simulink model "3_3PVstring"  (R2023b)
settings: Solver=ode3  StartTime=0.0  StopTime=1  FixedStep=1e-5  RelTol=1e-3
libraries: spsDiodeLib x18, spsPVArrayLib x9, spsIGBTDiodeLib x6, spsSeriesRLCBranchLib x3, spsSawtoothGeneratorLib x3, spsVoltageMeasurementLib x2, spsGroundLib x1, spsThreePhaseVIMeasurementLib x1, spsControlledVoltageSourceLib x1, spsCurrentMeasurementLib x1, simulink x1, sps_lib x1
settings Model: Creator=ameen  LastModifiedBy=safad

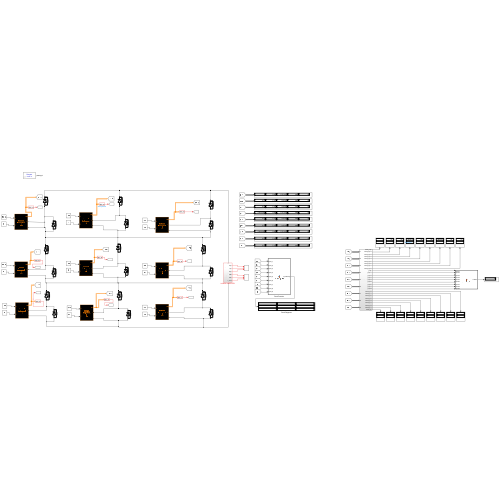
[thumbnail: Simulink's stored preview of the top-level diagram]
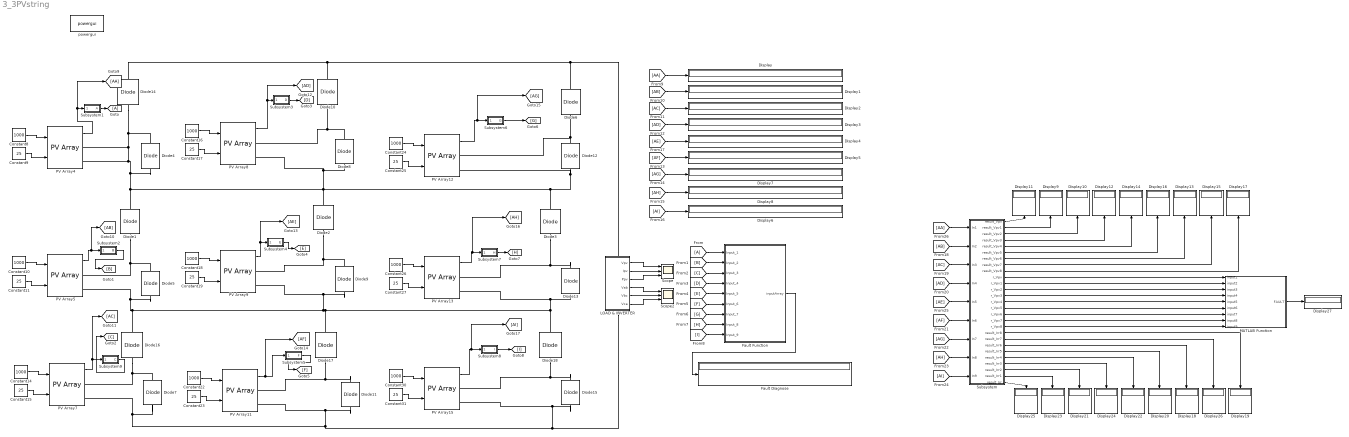
== system 3_3PVstring ==
  Constant{8,10,14,16,18,22,24,26,30} (9 alike) : Constant  Value=1000
  Constant{9,11,15,17,19,23,25,27,31} (9 alike) : Constant  Value=25
  Diode{1..18} (18 alike) : spsDiodeLib/Diode  Ron=0.001  Lon=0  Vf=0.8  IC=0  UseSnubber=0  Rs=500  Cs=250e-9  Measurements=off
  Display{,1..27} (28 alike) : Display
  Fault Diagnose : Display
  Fault Function : MATLAB Function  TreatAsAtomicUnit=on
  From : From
  Goto : Goto
  LOAD & INVERTER : Subsystem
      settings: PortSchema="{\"entries\":[{\"content\":{\"sides\":[{\"content\":{},\"type\":\"ConnectorPlacement.EquallySpacedRectSide\",\"uuid\":\"9d5a924a-1d3a-4741-a2b7-92be7c614fd7\"},{\"content\":{\"connectorIds\":[\"Out1\",\"Out2\",\"Out3\",\"Out4\",\"Out5\",\"Out6\"],\"side\":\"RIGHT\"},\"type\":\"ConnectorPlacement.EquallySpacedRectSide\",\"uuid\":\"42e89420-eace-4661-8437-77e02d17d38a\"},{\"content\":{\"connectorIds\":[\"LConn1\"],\"side\":\"TOP\"},\"type\":\"ConnectorPlacement.EquallySpacedRectSide\",\"uuid\":\"88a88f09-a234-44ff-a45c-243ed75cbb49\"},{\"content\":{\"connectorIds\":[\"RConn1\"],\"side\":\"BOTTOM\"},\"type\":\"ConnectorPlacement.EquallySpacedRectSide\",\"uuid\":\"b84592b4-f439-4f10-a620-72ac78255a9b\"}]},\"type\":\"ConnectorPlacement.EquallySpacedConnector\",\"uuid\":\"5a103a7e-397f-4ab8-8786-2dccd824124f\"}],\"packageUris\":[\"http://schema.mathworks.com/mf0/Connector/R2020b\"],\"version\":\"1.0\"}"
  MATLAB Function : MATLAB Function  TreatAsAtomicUnit=on
  PV Array{4..5,7..9,11..13,15} (9 alike) : spsPVArrayLib/PV Array  Npar=1  Nser=1  PlotType=array @ 25 deg.C & specified irradiances  S_vec="[ 1000  500  100 ]"  Temp_C_vec="[ 45 25  ]"  ModuleName=User-defined  PlotWhenSelected=off  Pm=213.15  Ncell=60  Voc=36.3  Isc=7.84  Vm=29  Im=7.35  beta_Voc_pc=-0.36099  alpha_Isc_pc=0.102  beta_Voc=-0.13104  alpha_Isc=0.0079968  IL=7.8654  I0=2.9273e-10  nI=0.98119  Rsh=313.0553  Rs=0.39381  RobustModel=off  RobustCellTemperature=313.3991  BAL=off  Tc=1e-6  Tfilter=1e-5
  Scope : Scope  NumInputPorts=3
  Scope2 : Scope  NumInputPorts=3
  Subsystem : Subsystem
  Subsystem1 : Subsystem
  Subsystem2 : Subsystem
  Subsystem3 : Subsystem
  Subsystem4 : Subsystem
  Subsystem5 : Subsystem
  Subsystem6 : Subsystem
  Subsystem7 : Subsystem
  Subsystem8 : Subsystem
  Subsystem9 : Subsystem
  powergui : sps_lib/powergui  Priority=1  SimulationMode=Discrete  SampleTime=1e-5  frequency=60  Iterations=50  frequencyindice=0  Pbase=100e6  ErrMax=1e-4  UnitsV=kV  UnitsW=MW  buscounter=0  FunctionMessages=off  echomessages=off  EnableUseOfTLC=off  CurrentSourceSwitches=off  DisableSnubberDevices=off  DisableRonSwitches=off  DisableVfSwitches=off  DisplayEquations=off  AutomaticDiscreteSolvers=off  SolverType=Tustin  Interpol=off  ExternalGateDelay=off  methode=off  Ts=100  x0status=blocks  SPID=on  SwTol=0  HookPort=off  NonlinearTolerance=1e-4  nMaxIteration=100  ContinueOnMaxIteration=off  RestoreLinks=warning  ResistiveCurrentMeasurement=off  Frange=[0:2:500]  Ylog=off  Xlog=on  ShowGrid=off  save=off  variable=ZData  structure=0  ZoomFFT=off  StartTime=0.0  cycles=1  DisplayStyle=1  fundamental=60  FreqAxis=off  MaxFrequency=1000  frequencyindicesteady=1  RmsSteady=1  display=off
  wires:
  Constant15/1 -> PV Array7/2
  Constant14/1 -> PV Array7/1
  Constant11/1 -> PV Array5/2
  Constant9/1 -> PV Array4/2
  Constant8/1 -> PV Array4/1
  Constant10/1 -> PV Array5/1
  Constant23/1 -> PV Array11/2
  Constant22/1 -> PV Array11/1
  Constant19/1 -> PV Array9/2
  Constant17/1 -> PV Array8/2
  Constant16/1 -> PV Array8/1
  Constant18/1 -> PV Array9/1
  Constant31/1 -> PV Array15/2
  Constant30/1 -> PV Array15/1
  Constant27/1 -> PV Array13/2
  Constant25/1 -> PV Array12/2
  Constant24/1 -> PV Array12/1
  Constant26/1 -> PV Array13/1
  PV Array4/1 -> [AA], Subsystem1/1(Vpv)
  Subsystem1/1(A) -> Goto/1
  Subsystem3/1(D) -> [D]
  PV Array8/1 -> [AD], Subsystem3/1(Vpv)
  PV Array12/1 -> [AG], Subsystem6/1(Vpv)
  Subsystem6/1(G) -> [G]
  Subsystem2/1(B) -> [B]
  PV Array5/1 -> [AB], Subsystem2/1(Vpv)
  PV Array9/1 -> [AE], Subsystem4/1(Vpv)
  Subsystem4/1(E) -> [E]
  Subsystem5/1(F) -> [F]
  PV Array11/1 -> [AF], Subsystem5/1(Vpv)
  Subsystem7/1(H) -> [H]
  PV Array13/1 -> [AH], Subsystem7/1(Vpv)
  Subsystem8/1(I) -> [I]
  PV Array15/1 -> [AI], Subsystem8/1(Vpv)
  [D] -> Fault Function/4(Input_4)
  [B] -> Fault Function/2(Input_2)
  [F] -> Fault Function/6(Input_6)
  [E] -> Fault Function/5(Input_5)
  [G] -> Fault Function/7(Input_7)
  Fault Function/1(inputArray) -> Fault Diagnose/1
  [C] -> Fault Function/3(Input_3)
  [I] -> Fault Function/9(Input_9)
  [H] -> Fault Function/8(Input_8)
  From/1 -> Fault Function/1(Input_1)
  PV Array7/1 -> [AC], Subsystem9/1(Vpv)
  Subsystem9/1(C) -> [C]
  LOAD & INVERTER/1(Vpv) -> Scope/1
  LOAD & INVERTER/2(Ipv) -> Scope/2
  LOAD & INVERTER/3(Ppv) -> Scope/3
  LOAD & INVERTER/4(Vab) -> Scope2/1
  LOAD & INVERTER/5(Vbc) -> Scope2/2
  LOAD & INVERTER/6(Vca) -> Scope2/3
  [AA] -> Display/1
  [AB] -> Display1/1
  [AC] -> Display2/1
  [AD] -> Display3/1
  [AE] -> Display4/1
  [AF] -> Display5/1
  [AG] -> Display7/1
  [AH] -> Display8/1
  [AI] -> Display6/1
  [AA] -> Subsystem/1(In1)
  [AB] -> Subsystem/2(In2)
  [AC] -> Subsystem/3(In3)
  [AD] -> Subsystem/4(In4)
  [AE] -> Subsystem/5(In5)
  [AF] -> Subsystem/6(In6)
  [AG] -> Subsystem/7(In7)
  [AH] -> Subsystem/8(In8)
  [AI] -> Subsystem/9(In9)
  Subsystem/1(result_Vpv) -> Display11/1
  Subsystem/2(result_Vpv1) -> Display9/1
  Subsystem/3(result_Vpv2) -> Display10/1
  Subsystem/4(result_Vpv3) -> Display12/1
  Subsystem/5(result_Vpv4) -> Display14/1
  Subsystem/6(result_Vpv5) -> Display16/1
  Subsystem/7(result_Vpv6) -> Display13/1
  Subsystem/8(result_Vpv7) -> Display15/1
  Subsystem/9(result_Vpv8) -> Display17/1
  Subsystem/27(result_Irr) -> Display25/1
  Subsystem/26(result_Irr1) -> Display23/1
  Subsystem/25(result_Irr2) -> Display21/1
  Subsystem/24(result_Irr3) -> Display24/1
  Subsystem/23(result_Irr4) -> Display22/1
  Subsystem/22(result_Irr5) -> Display20/1
  Subsystem/21(result_Irr6) -> Display18/1
  Subsystem/20(result_Irr7) -> Display26/1
  Subsystem/19(result_Irr8) -> Display19/1
  Subsystem/10(r_Vpv) -> MATLAB Function/1(input1)
  Subsystem/11(r_Vpv1) -> MATLAB Function/2(input2)
  Subsystem/12(r_Vpv2) -> MATLAB Function/3(input3)
  Subsystem/13(r_Vpv3) -> MATLAB Function/4(input4)
  Subsystem/14(r_Vpv4) -> MATLAB Function/5(input5)
  Subsystem/15(r_Vpv5) -> MATLAB Function/6(input6)
  Subsystem/16(r_Vpv6) -> MATLAB Function/7(input7)
  Subsystem/17(r_Vpv7) -> MATLAB Function/8(input8)
  Subsystem/18(r_Vpv8) -> MATLAB Function/9(input9)
  MATLAB Function/1(FAULT) -> Display27/1
  connections:
  Diode13/RConn1 -- Diode3/LConn1 -- PV Array13/RConn1
  Diode8/RConn1 -- Diode10/LConn1 -- PV Array8/RConn1
  Diode9/LConn1 -- Diode5/LConn1 -- PV Array5/RConn2 -- Diode16/RConn1 -- Diode17/RConn1 -- Diode13/LConn1 -- PV Array13/RConn2 -- Diode18/RConn1 -- PV Array9/RConn2
  Diode15/RConn1 -- Diode18/LConn1 -- PV Array15/RConn1
  Diode11/RConn1 -- Diode17/LConn1 -- PV Array11/RConn1
  Diode10/RConn1 -- Diode14/RConn1 -- Diode6/RConn1 -- LOAD & INVERTER/LConn1
  Diode1/LConn1 -- Diode5/RConn1 -- PV Array5/RConn1
  Diode16/LConn1 -- Diode7/RConn1 -- PV Array7/RConn1
  Diode12/RConn1 -- Diode6/LConn1 -- PV Array12/RConn1
  Diode11/LConn1 -- Diode7/LConn1 -- PV Array7/RConn2 -- LOAD & INVERTER/RConn1 -- Diode15/LConn1 -- PV Array15/RConn2 -- PV Array11/RConn2
  Diode9/RConn1 -- Diode2/LConn1 -- PV Array9/RConn1
  Diode14/LConn1 -- Diode4/RConn1 -- PV Array4/RConn2 -- Diode4/LConn1 -- Diode8/LConn1 -- PV Array8/RConn2 -- Diode2/RConn1 -- Diode12/LConn1 -- PV Array12/RConn2 -- Diode3/RConn1 -- Diode1/RConn1 -- PV Array4/RConn1

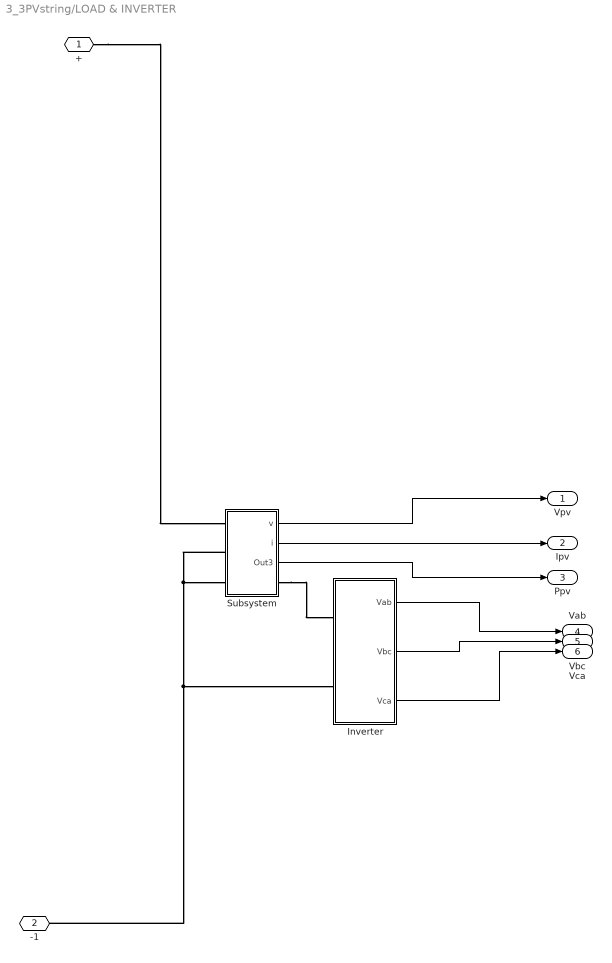
== system 3_3PVstring/LOAD & INVERTER ==
  Inverter : Subsystem
  Subsystem : Subsystem
  + : PMIOPort  Side=Left
  -1 : PMIOPort  Port=2  Side=Right
  Vpv : Outport
  Ipv : Outport  Port=2
  Ppv : Outport  Port=3
  Vab : Outport  Port=4
  Vbc : Outport  Port=5
  Vca : Outport  Port=6
  wires:
  Subsystem/1(v) -> Vpv/1
  Subsystem/2(i) -> Ipv/1
  Subsystem/3(Out3) -> Ppv/1
  Inverter/1(Vab) -> Vab/1
  Inverter/2(Vbc) -> Vbc/1
  Inverter/3(Vca) -> Vca/1
  connections:
  Subsystem/RConn1 -- Inverter/LConn1
  Subsystem/LConn2 -- -1/RConn1 -- Inverter/LConn2 -- Subsystem/LConn3
  +/RConn1 -- Subsystem/LConn1

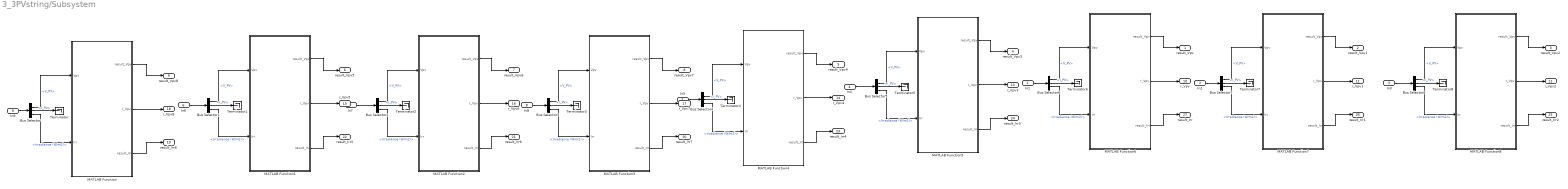
== system 3_3PVstring/Subsystem ==
  In1 : Inport
  In2 : Inport  Port=2
  In3 : Inport  Port=3
  In4 : Inport  Port=4
  In5 : Inport  Port=5
  In6 : Inport  Port=6
  In7 : Inport  Port=7
  In8 : Inport  Port=8
  In9 : Inport  Port=9
  Bus Selector{,1..8} (9 alike) : BusSelector  OutputSignals=V_PV,I_PV,Irradiance (W/m2)
  MATLAB Function : MATLAB Function  TreatAsAtomicUnit=on
  MATLAB Function1 : MATLAB Function  TreatAsAtomicUnit=on
  MATLAB Function2 : MATLAB Function  TreatAsAtomicUnit=on
  MATLAB Function3 : MATLAB Function  TreatAsAtomicUnit=on
  MATLAB Function4 : MATLAB Function  TreatAsAtomicUnit=on
  MATLAB Function5 : MATLAB Function  TreatAsAtomicUnit=on
  MATLAB Function6 : MATLAB Function  TreatAsAtomicUnit=on
  MATLAB Function7 : MATLAB Function  TreatAsAtomicUnit=on
  MATLAB Function8 : MATLAB Function  TreatAsAtomicUnit=on
  Terminator{,1..8} (9 alike) : Terminator
  result_Vpv : Outport
  result_Vpv1 : Outport  Port=2
  result_Vpv2 : Outport  Port=3
  result_Vpv3 : Outport  Port=4
  result_Vpv4 : Outport  Port=5
  result_Vpv5 : Outport  Port=6
  result_Vpv6 : Outport  Port=7
  result_Vpv7 : Outport  Port=8
  result_Vpv8 : Outport  Port=9
  r_Vpv : Outport  Port=10
  r_Vpv1 : Outport  Port=11
  r_Vpv2 : Outport  Port=12
  r_Vpv3 : Outport  Port=13
  r_Vpv4 : Outport  Port=14
  r_Vpv5 : Outport  Port=15
  r_Vpv6 : Outport  Port=16
  r_Vpv7 : Outport  Port=17
  r_Vpv8 : Outport  Port=18
  result_Irr8 : Outport  Port=19
  result_Irr7 : Outport  Port=20
  result_Irr6 : Outport  Port=21
  result_Irr5 : Outport  Port=22
  result_Irr4 : Outport  Port=23
  result_Irr3 : Outport  Port=24
  result_Irr2 : Outport  Port=25
  result_Irr1 : Outport  Port=26
  result_Irr : Outport  Port=27
  wires:
  MATLAB Function7/1(result_Vpv) -> result_Vpv1/1
  Bus Selector6/2 -> Terminator6/1  "<I_PV>"
  In3/1 -> Bus Selector8/1
  Bus Selector6/1 -> MATLAB Function6/1(Vpv)  "<V_PV>"
  Bus Selector/3 -> MATLAB Function/2(Irr)  "<Irradiance (W/m2)>"
  MATLAB Function8/1(result_Vpv) -> result_Vpv2/1
  Bus Selector1/3 -> MATLAB Function1/2(Irr)  "<Irradiance (W/m2)>"
  Bus Selector/1 -> MATLAB Function/1(Vpv)  "<V_PV>"
  MATLAB Function3/1(result_Vpv) -> result_Vpv7/1
  MATLAB Function8/2(r_Vpv) -> r_Vpv2/1
  In7/1 -> Bus Selector2/1
  MATLAB Function2/1(result_Vpv) -> result_Vpv6/1
  MATLAB Function6/1(result_Vpv) -> result_Vpv/1
  Bus Selector/2 -> Terminator/1  "<I_PV>"
  Bus Selector7/1 -> MATLAB Function7/1(Vpv)  "<V_PV>"
  MATLAB Function3/3(result_Irr) -> result_Irr7/1
  Bus Selector2/2 -> Terminator2/1  "<I_PV>"
  Bus Selector6/3 -> MATLAB Function6/2(Irr)  "<Irradiance (W/m2)>"
  In4/1 -> Bus Selector5/1
  MATLAB Function6/3(result_Irr) -> result_Irr/1
  MATLAB Function7/3(result_Irr) -> result_Irr1/1
  MATLAB Function/2(r_Vpv) -> r_Vpv8/1
  Bus Selector1/1 -> MATLAB Function1/1(Vpv)  "<V_PV>"
  Bus Selector7/3 -> MATLAB Function7/2(Irr)  "<Irradiance (W/m2)>"
  MATLAB Function5/3(result_Irr) -> result_Irr3/1
  Bus Selector4/3 -> MATLAB Function4/2(Irr)  "<Irradiance (W/m2)>"
  MATLAB Function1/2(r_Vpv) -> r_Vpv5/1
  MATLAB Function2/2(r_Vpv) -> r_Vpv6/1
  Bus Selector1/2 -> Terminator1/1  "<I_PV>"
  MATLAB Function3/2(r_Vpv) -> r_Vpv7/1
  Bus Selector3/2 -> Terminator3/1  "<I_PV>"
  In8/1 -> Bus Selector3/1
  Bus Selector3/1 -> MATLAB Function3/1(Vpv)  "<V_PV>"
  MATLAB Function8/3(result_Irr) -> result_Irr2/1
  Bus Selector3/3 -> MATLAB Function3/2(Irr)  "<Irradiance (W/m2)>"
  Bus Selector7/2 -> Terminator7/1  "<I_PV>"
  Bus Selector4/2 -> Terminator4/1  "<I_PV>"
  MATLAB Function2/3(result_Irr) -> result_Irr6/1
  MATLAB Function5/1(result_Vpv) -> result_Vpv3/1
  Bus Selector4/1 -> MATLAB Function4/1(Vpv)  "<V_PV>"
  Bus Selector2/3 -> MATLAB Function2/2(Irr)  "<Irradiance (W/m2)>"
  In1/1 -> Bus Selector6/1
  Bus Selector5/2 -> Terminator5/1  "<I_PV>"
  Bus Selector8/2 -> Terminator8/1  "<I_PV>"
  Bus Selector2/1 -> MATLAB Function2/1(Vpv)  "<V_PV>"
  In5/1 -> Bus Selector4/1
  Bus Selector8/1 -> MATLAB Function8/1(Vpv)  "<V_PV>"
  Bus Selector8/3 -> MATLAB Function8/2(Irr)  "<Irradiance (W/m2)>"
  In6/1 -> Bus Selector1/1
  MATLAB Function6/2(r_Vpv) -> r_Vpv/1
  MATLAB Function4/1(result_Vpv) -> result_Vpv4/1
  Bus Selector5/3 -> MATLAB Function5/2(Irr)  "<Irradiance (W/m2)>"
  MATLAB Function5/2(r_Vpv) -> r_Vpv3/1
  Bus Selector5/1 -> MATLAB Function5/1(Vpv)  "<V_PV>"
  MATLAB Function/3(result_Irr) -> result_Irr8/1
  MATLAB Function1/3(result_Irr) -> result_Irr5/1
  In9/1 -> Bus Selector/1
  MATLAB Function/1(result_Vpv) -> result_Vpv8/1
  MATLAB Function1/1(result_Vpv) -> result_Vpv5/1
  In2/1 -> Bus Selector7/1
  MATLAB Function7/2(r_Vpv) -> r_Vpv1/1
  MATLAB Function4/2(r_Vpv) -> r_Vpv4/1
  MATLAB Function4/3(result_Irr) -> result_Irr4/1

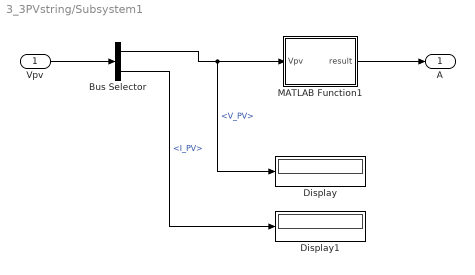
== system 3_3PVstring/Subsystem1 ==
  Vpv : Inport
  Bus Selector : BusSelector  OutputSignals=V_PV,I_PV
  Display : Display
  Display1 : Display
  MATLAB Function1 : MATLAB Function  TreatAsAtomicUnit=on
  A : Outport
  wires:
  Vpv/1 -> Bus Selector/1
  MATLAB Function1/1(result) -> A/1
  Bus Selector/1 -> Display/1, MATLAB Function1/1(Vpv)  "<V_PV>"
  Bus Selector/2 -> Display1/1  "<I_PV>"

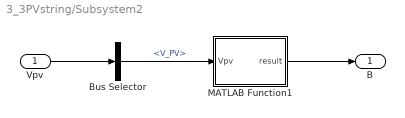
== system 3_3PVstring/Subsystem2 ==
  Vpv : Inport
  Bus Selector : BusSelector  OutputSignals=V_PV
  MATLAB Function1 : MATLAB Function  TreatAsAtomicUnit=on
  B : Outport
  wires:
  MATLAB Function1/1(result) -> B/1
  Vpv/1 -> Bus Selector/1
  Bus Selector/1 -> MATLAB Function1/1(Vpv)  "<V_PV>"

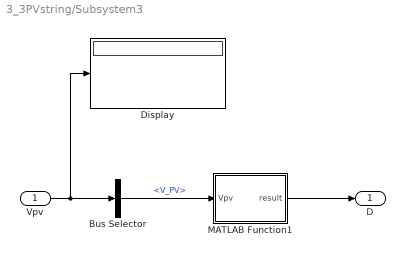
== system 3_3PVstring/Subsystem3 ==
  Vpv : Inport
  Bus Selector : BusSelector  OutputSignals=V_PV
  Display : Display
  MATLAB Function1 : MATLAB Function  TreatAsAtomicUnit=on
  D : Outport
  wires:
  MATLAB Function1/1(result) -> D/1
  Vpv/1 -> Bus Selector/1, Display/1
  Bus Selector/1 -> MATLAB Function1/1(Vpv)  "<V_PV>"

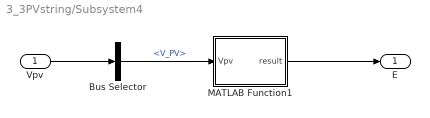
== system 3_3PVstring/Subsystem4 ==
  Vpv : Inport
  Bus Selector : BusSelector  OutputSignals=V_PV
  MATLAB Function1 : MATLAB Function  TreatAsAtomicUnit=on
  E : Outport
  wires:
  Bus Selector/1 -> MATLAB Function1/1(Vpv)  "<V_PV>"
  Vpv/1 -> Bus Selector/1
  MATLAB Function1/1(result) -> E/1

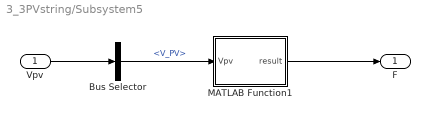
== system 3_3PVstring/Subsystem5 ==
  Vpv : Inport
  Bus Selector : BusSelector  OutputSignals=V_PV
  MATLAB Function1 : MATLAB Function  TreatAsAtomicUnit=on
  F : Outport
  wires:
  MATLAB Function1/1(result) -> F/1
  Vpv/1 -> Bus Selector/1
  Bus Selector/1 -> MATLAB Function1/1(Vpv)  "<V_PV>"

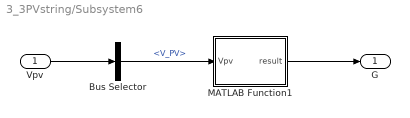
== system 3_3PVstring/Subsystem6 ==
  Vpv : Inport
  Bus Selector : BusSelector  OutputSignals=V_PV
  MATLAB Function1 : MATLAB Function  TreatAsAtomicUnit=on
  G : Outport
  wires:
  Bus Selector/1 -> MATLAB Function1/1(Vpv)  "<V_PV>"
  Vpv/1 -> Bus Selector/1
  MATLAB Function1/1(result) -> G/1

== system 3_3PVstring/Subsystem7 ==
  Vpv : Inport
  Bus Selector : BusSelector  OutputSignals=V_PV
  MATLAB Function1 : MATLAB Function  TreatAsAtomicUnit=on
  H : Outport
  wires:
  MATLAB Function1/1(result) -> H/1
  Vpv/1 -> Bus Selector/1
  Bus Selector/1 -> MATLAB Function1/1(Vpv)  "<V_PV>"

== system 3_3PVstring/Subsystem8 ==
  Vpv : Inport
  Bus Selector : BusSelector  OutputSignals=V_PV
  MATLAB Function1 : MATLAB Function  TreatAsAtomicUnit=on
  I : Outport
  wires:
  Bus Selector/1 -> MATLAB Function1/1(Vpv)  "<V_PV>"
  Vpv/1 -> Bus Selector/1
  MATLAB Function1/1(result) -> I/1

== system 3_3PVstring/Subsystem9 ==
  Vpv : Inport
  Bus Selector : BusSelector  OutputSignals=V_PV
  MATLAB Function1 : MATLAB Function  TreatAsAtomicUnit=on
  C : Outport
  wires:
  Bus Selector/1 -> MATLAB Function1/1(Vpv)  "<V_PV>"
  Vpv/1 -> Bus Selector/1
  MATLAB Function1/1(result) -> C/1

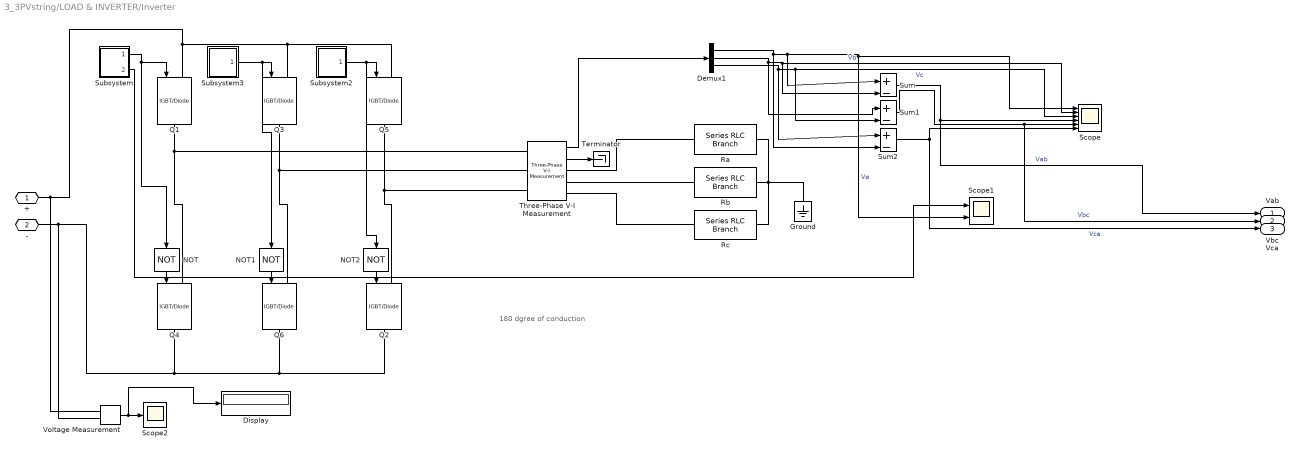
== system 3_3PVstring/LOAD & INVERTER/Inverter ==
  note: 180 dgree of conduction
  Demux1 : Demux  Outputs=3
  Display : Display
  Ground : spsGroundLib/Ground  LConnTagsString=a
  NOT : Logic  Operator=NOT  AllPortsSameDT=off  OutDataTypeStr=boolean
  NOT1 : Logic  Operator=NOT  AllPortsSameDT=off  OutDataTypeStr=boolean
  NOT2 : Logic  Operator=NOT  AllPortsSameDT=off  OutDataTypeStr=boolean
  Q{1..6} (6 alike) : spsIGBTDiodeLib/IGBT//Diode  Ron=1e-3  Rs=1e5  Cs=inf  Measurements=off
  Ra : spsSeriesRLCBranchLib/Series RLC Branch  LConnTagsString=__new0  RConnTagsString=__new0  BranchType=R  Resistance=-0.5820  Inductance=1e-3  SetiL0=off  InitialCurrent=0  Capacitance=1e-6  Setx0=off  InitialVoltage=0  Measurements=None
  Rb : spsSeriesRLCBranchLib/Series RLC Branch  LConnTagsString=__new0  RConnTagsString=__new0  BranchType=R  Resistance=1  Inductance=1e-3  SetiL0=off  InitialCurrent=0  Capacitance=1e-6  Setx0=off  InitialVoltage=0  Measurements=None
  Rc : spsSeriesRLCBranchLib/Series RLC Branch  LConnTagsString=__new0  RConnTagsString=__new0  BranchType=R  Resistance=1  Inductance=1e-3  SetiL0=off  InitialCurrent=0  Capacitance=1e-6  Setx0=off  InitialVoltage=0  Measurements=None
  Scope : Scope  NumInputPorts=6
  Scope1 : Scope  NumInputPorts=2
  Scope2 : Scope
  Subsystem : Subsystem
  Subsystem2 : Subsystem
  Subsystem3 : Subsystem
  Sum : Sum  Inputs=|+-
  Sum1 : Sum  Inputs=|+-
  Sum2 : Sum  Inputs=|+-
  Terminator : Terminator
  Three-Phase V-I Measurement : spsThreePhaseVIMeasurementLib/Three-Phase V-I Measurement  VoltageMeasurement=phase-to-ground  SetLabelV=off  LabelV=Vabc  Vpu=off  VpuLL=off  CurrentMeasurement=yes  SetLabelI=off  LabelI=Iabc  Ipu=off  Pbase=100e6  Vbase=500e3  OutputType=Complex  PhasorSimulation=off  PSBequivalent=0
  Voltage Measurement : spsVoltageMeasurementLib/Voltage Measurement  PhasorSimulation=off  OutputType=Complex  PSBequivalent=0
  + : PMIOPort  Side=Left
  - : PMIOPort  Port=2  Side=Left
  Vab : Outport
  Vbc : Outport  Port=2
  Vca : Outport  Port=3
  wires:
  Sum2/1 -> Vca/1, Scope/6  "Vca"
  Subsystem/2(Outport) -> Scope1/1
  Sum1/1 -> Vbc/1, Scope/5  "Vbc"
  Three-Phase V-I Measurement/1 -> Demux1/1
  Sum/1 -> Vab/1, Scope/4  "Vab"
  Subsystem/1(Out1) -> NOT/1, Q1/1
  Three-Phase V-I Measurement/2 -> Terminator/1
  NOT/1 -> Q4/1
  Subsystem3/1(Out1) -> Q3/1, NOT1/1
  Subsystem2/1(Out1) -> Q5/1, NOT2/1
  Demux1/3 -> Sum2/1, Sum1/2, Scope/3  "Vc"
  Demux1/2 -> Sum1/1, Sum/2, Scope/2  "Vb"
  NOT2/1 -> Q2/1
  NOT1/1 -> Q6/1
  Demux1/1 -> Sum2/2, Sum/1, Scope1/2, Scope/1  "Va"
  Voltage Measurement/1 -> Display/1, Scope2/1
  connections:
  Three-Phase V-I Measurement/LConn1 -- Q4/LConn1 -- Q1/RConn1
  Three-Phase V-I Measurement/LConn2 -- Q6/LConn1 -- Q3/RConn1
  Q1/LConn1 -- Voltage Measurement/LConn1 -- +/RConn1 -- Q3/LConn1 -- Q5/LConn1
  Q4/RConn1 -- Voltage Measurement/LConn2 -- -/RConn1 -- Q2/RConn1 -- Q6/RConn1
  Three-Phase V-I Measurement/LConn3 -- Q2/LConn1 -- Q5/RConn1
  Ground/LConn1 -- Ra/RConn1 -- Rc/RConn1 -- Rb/RConn1
  Rc/LConn1 -- Three-Phase V-I Measurement/RConn3
  Ra/LConn1 -- Three-Phase V-I Measurement/RConn1
  Rb/LConn1 -- Three-Phase V-I Measurement/RConn2

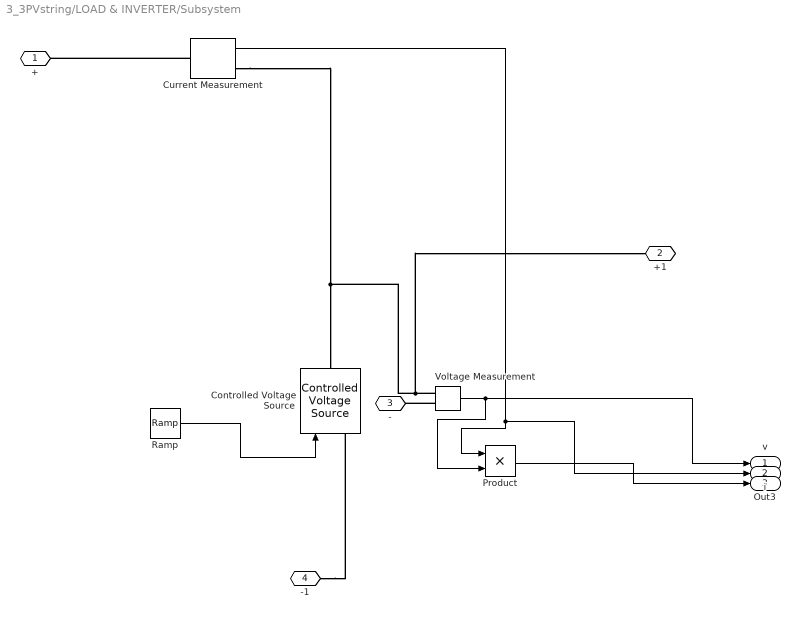
== system 3_3PVstring/LOAD & INVERTER/Subsystem ==
  Controlled Voltage Source : spsControlledVoltageSourceLib/Controlled Voltage Source  Initialize=on  Source_Type=AC  Amplitude=0  Phase=0  Frequency=0  Measurements=None
  Current Measurement : spsCurrentMeasurementLib/Current Measurement  PhasorSimulation=off  OutputType=Complex  PSBequivalent=0
  Product : Product
  Ramp : simulink/Sources/Ramp  slope=36.3*3  start=0  InitialOutput=0
  Voltage Measurement : spsVoltageMeasurementLib/Voltage Measurement  PhasorSimulation=off  OutputType=Complex  PSBequivalent=0
  + : PMIOPort  Side=Left
  +1 : PMIOPort  Port=2  Side=Right
  - : PMIOPort  Port=3  Side=Left
  -1 : PMIOPort  Port=4  Side=Left
  v : Outport
  i : Outport  Port=2
  Out3 : Outport  Port=3
  wires:
  Current Measurement/1 -> i/1, Product/1
  Ramp/1 -> Controlled Voltage Source/1
  Voltage Measurement/1 -> v/1, Product/2
  Product/1 -> Out3/1
  connections:
  Current Measurement/LConn1 -- +/RConn1
  Current Measurement/RConn1 -- +1/RConn1 -- Voltage Measurement/LConn1 -- Controlled Voltage Source/RConn1
  Voltage Measurement/LConn2 -- -/RConn1
  -1/RConn1 -- Controlled Voltage Source/LConn1

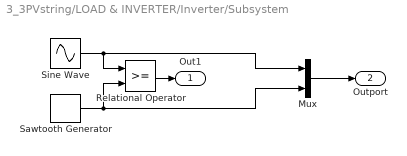
== system 3_3PVstring/LOAD & INVERTER/Inverter/Subsystem ==
  Mux : Mux  Inputs=2
  Relational Operator : RelationalOperator  OutDataTypeStr=boolean  RndMeth=Simplest  InputSameDT=off
  Sawtooth Generator : spsSawtoothGeneratorLib/Sawtooth Generator  Freq=1e3  Phase=180  Ts=0
  Sine Wave : Sin  Amplitude=0.9  Frequency=2*pi*50  SampleTime=0
  Out1 : Outport
  Outport : Outport  Port=2
  wires:
  Sine Wave/1 -> Mux/1, Relational Operator/1
  Relational Operator/1 -> Out1/1
  Sawtooth Generator/1 -> Mux/2, Relational Operator/2
  Mux/1 -> Outport/1

== system 3_3PVstring/LOAD & INVERTER/Inverter/Subsystem2 ==
  Relational Operator : RelationalOperator  OutDataTypeStr=boolean  RndMeth=Simplest  InputSameDT=off
  Sawtooth Generator : spsSawtoothGeneratorLib/Sawtooth Generator  Freq=1e3  Phase=180  Ts=0
  Sine Wave : Sin  Amplitude=0.9  Frequency=2*pi*50  Phase=240*pi/180  SampleTime=0
  Out1 : Outport
  wires:
  Sine Wave/1 -> Relational Operator/1
  Relational Operator/1 -> Out1/1
  Sawtooth Generator/1 -> Relational Operator/2

== system 3_3PVstring/LOAD & INVERTER/Inverter/Subsystem3 ==
  Relational Operator : RelationalOperator  OutDataTypeStr=boolean  RndMeth=Simplest  InputSameDT=off
  Sawtooth Generator : spsSawtoothGeneratorLib/Sawtooth Generator  Freq=1e3  Phase=180  Ts=0
  Sine Wave : Sin  Amplitude=0.9  Frequency=2*pi*50  Phase=120*pi/180  SampleTime=0
  Out1 : Outport
  wires:
  Sine Wave/1 -> Relational Operator/1
  Relational Operator/1 -> Out1/1
  Sawtooth Generator/1 -> Relational Operator/2

== matlab function 3_3PVstring/Subsystem/MATLAB Function ==
  data: Vpv input; Irr input; result_Vpv output; r_Vpv output; result_Irr output
function [result_Vpv, r_Vpv, result_Irr] = checkValues(Vpv, Irr)
    % Check Vpv
    if Vpv < 35
        result_Vpv = [Vpv, 1];  % Output Vpv value and 1
        r_Vpv = 1;
        disp('SC or LL');
    else
        result_Vpv = [0, 0];    % Output 0 and 0
        r_Vpv = 0;
    end

    % Check Irr
    if Irr < 1000
        result_Irr = [Irr, 1];  % Output Irr value and 1
        disp('Partial Shading');
    else
        result_Irr = [0, 0];    % Output 0 and 0
    end
end

== matlab function 3_3PVstring/Subsystem/MATLAB Function1 ==
  data: Vpv input; Irr input; result_Vpv output; r_Vpv output; result_Irr output
function [result_Vpv, r_Vpv, result_Irr] = checkValues(Vpv, Irr)
    % Check Vpv
    if Vpv < 35
        result_Vpv = [Vpv, 1];  % Output Vpv value and 1
        r_Vpv = 1;
        disp('SC or LL');
    else
        result_Vpv = [0, 0];    % Output 0 and 0
        r_Vpv = 0;
    end

    % Check Irr
    if Irr < 1000
        result_Irr = [Irr, 1];  % Output Irr value and 1
        disp('Partial Shading');
    else
        result_Irr = [0, 0];    % Output 0 and 0
    end
end

== matlab function 3_3PVstring/Subsystem/MATLAB Function2 ==
  data: Vpv input; Irr input; result_Vpv output; r_Vpv output; result_Irr output
function [result_Vpv, r_Vpv, result_Irr] = checkValues(Vpv, Irr)
    % Check Vpv
    if Vpv < 35
        result_Vpv = [Vpv, 1];  % Output Vpv value and 1
        r_Vpv = 1;
        disp('SC or LL');
    else
        result_Vpv = [0, 0];    % Output 0 and 0
        r_Vpv = 0;
    end

    % Check Irr
    if Irr < 1000
        result_Irr = [Irr, 1];  % Output Irr value and 1
        disp('Partial Shading');
    else
        result_Irr = [0, 0];    % Output 0 and 0
    end
end

== matlab function 3_3PVstring/Subsystem/MATLAB Function3 ==
  data: Vpv input; Irr input; result_Vpv output; r_Vpv output; result_Irr output
function [result_Vpv, r_Vpv, result_Irr] = checkValues(Vpv, Irr)
    % Check Vpv
    if Vpv < 35
        result_Vpv = [Vpv, 1];  % Output Vpv value and 1
        r_Vpv = 1;
        disp('SC or LL');
    else
        result_Vpv = [0, 0];    % Output 0 and 0
        r_Vpv = 0;
    end

    % Check Irr
    if Irr < 1000
        result_Irr = [Irr, 1];  % Output Irr value and 1
        disp('Partial Shading');
    else
        result_Irr = [0, 0];    % Output 0 and 0
    end
end

== matlab function 3_3PVstring/Subsystem/MATLAB Function4 ==
  data: Vpv input; Irr input; result_Vpv output; r_Vpv output; result_Irr output
function [result_Vpv, r_Vpv, result_Irr] = checkValues(Vpv, Irr)
    % Check Vpv
    if Vpv < 35
        result_Vpv = [Vpv, 1];  % Output Vpv value and 1
        r_Vpv = 1;
        disp('SC or LL');
    else
        result_Vpv = [0, 0];    % Output 0 and 0
        r_Vpv = 0;
    end

    % Check Irr
    if Irr < 1000
        result_Irr = [Irr, 1];  % Output Irr value and 1
        disp('Partial Shading');
    else
        result_Irr = [0, 0];    % Output 0 and 0
    end
end

== matlab function 3_3PVstring/Subsystem/MATLAB Function5 ==
  data: Vpv input; Irr input; result_Vpv output; r_Vpv output; result_Irr output
function [result_Vpv, r_Vpv, result_Irr] = checkValues(Vpv, Irr)
    % Check Vpv
    if Vpv < 35
        result_Vpv = [Vpv, 1];  % Output Vpv value and 1
        r_Vpv = 1;
        disp('SC or LL');
    else
        result_Vpv = [0, 0];    % Output 0 and 0
        r_Vpv = 0;
    end

    % Check Irr
    if Irr < 1000
        result_Irr = [Irr, 1];  % Output Irr value and 1
        disp('Partial Shading');
    else
        result_Irr = [0, 0];    % Output 0 and 0
    end
end

== matlab function 3_3PVstring/Subsystem/MATLAB Function6 ==
  data: Vpv input; Irr input; result_Vpv output; r_Vpv output; result_Irr output
function [result_Vpv, r_Vpv, result_Irr] = checkValues(Vpv, Irr)
    % Check Vpv
    if Vpv < 35
        result_Vpv = [Vpv, 1];  % Output Vpv value and 1
        r_Vpv = 1;
        disp('SC or LL');
    else
        result_Vpv = [0, 0];    % Output 0 and 0
        r_Vpv = 0;
    end

    % Check Irr
    if Irr < 1000
        result_Irr = [Irr, 1];  % Output Irr value and 1
        disp('Partial Shading');
    else
        result_Irr = [0, 0];    % Output 0 and 0
    end
end

== matlab function 3_3PVstring/Subsystem/MATLAB Function7 ==
  data: Vpv input; Irr input; result_Vpv output; r_Vpv output; result_Irr output
function [result_Vpv, r_Vpv, result_Irr] = checkValues(Vpv, Irr)
    % Check Vpv
    if Vpv < 35
        result_Vpv = [Vpv, 1];  % Output Vpv value and 1
        r_Vpv = 1;
        disp('SC or LL');
    else
        result_Vpv = [0, 0];    % Output 0 and 0
        r_Vpv = 0;
    end

    % Check Irr
    if Irr < 1000
        result_Irr = [Irr, 1];  % Output Irr value and 1
        disp('Partial Shading');
    else
        result_Irr = [0, 0];    % Output 0 and 0
    end
end

== matlab function 3_3PVstring/Subsystem/MATLAB Function8 ==
  data: Vpv input; Irr input; result_Vpv output; r_Vpv output; result_Irr output
function [result_Vpv, r_Vpv, result_Irr] = checkValues(Vpv, Irr)
    % Check Vpv
    if Vpv < 35
        result_Vpv = [Vpv, 1];  % Output Vpv value and 1
        r_Vpv = 1;
        disp('SC or LL');
    else
        result_Vpv = [0, 0];    % Output 0 and 0
        r_Vpv = 0;
    end

    % Check Irr
    if Irr < 1000
        result_Irr = [Irr, 1];  % Output Irr value and 1
        disp('Partial Shading');
    else
        result_Irr = [0, 0];    % Output 0 and 0
    end
end

== matlab function 3_3PVstring/MATLAB Function ==
  data: input1 input; input2 input; input3 input; input4 input; input5 input; input6 input; input7 input; input8 input; input9 input; FAULT output
function FAULT  = checkFaults(input1, input2, input3, input4, input5, input6, input7, input8, input9)
    % Count how many inputs are equal to 1
    countOnes = sum([input1, input2, input3, input4, input5, input6, input7, input8, input9] == 1);

    % Check the number of inputs equal to 1
    if countOnes > 1
        disp('LL or LG or LLG Fault');
        FAULT = 10;
    else
        disp('SC Fault');
        FAULT = 100;
    end
end

== matlab function 3_3PVstring/Subsystem1/MATLAB Function1 ==
  data: Vpv input; result output
function result = checkVpv(Vpv)
    if Vpv == 0
        result = 1;
    else
        result = 0;
    end
end

== matlab function 3_3PVstring/Fault Function ==
  data: Input_1 input; inputArray output; Input_2 input; Input_3 input; Input_4 input; Input_5 input; Input_6 input; Input_7 input; Input_8 input; Input_9 input
function inputArray = collectInputs(Input_1, Input_2, Input_3, Input_4, Input_5, Input_6, Input_7, Input_8, Input_9)
    % Create an array to store the 9 input values
    inputArray = [Input_1, Input_4, Input_7, Input_2, Input_5, Input_6, Input_3, Input_8, Input_9];
end

== matlab function 3_3PVstring/Subsystem2/MATLAB Function1 ==
  data: Vpv input; result output
function result = checkVpv(Vpv)
    if Vpv == 0
        result = 1;
    else
        result = 0;
    end
end

== matlab function 3_3PVstring/Subsystem9/MATLAB Function1 ==
  data: Vpv input; result output
function result = checkVpv(Vpv)
    if Vpv == 0
        result = 1;
    else
        result = 0;
    end
end

== matlab function 3_3PVstring/Subsystem3/MATLAB Function1 ==
  data: Vpv input; result output
function result = checkVpv(Vpv)
    if Vpv == 0
        result = 1;
    else
        result = 0;
    end
end

== matlab function 3_3PVstring/Subsystem4/MATLAB Function1 ==
  data: Vpv input; result output
function result = checkVpv(Vpv)
    if Vpv == 0
        result = 1;
    else
        result = 0;
    end
end

== matlab function 3_3PVstring/Subsystem5/MATLAB Function1 ==
  data: Vpv input; result output
function result = checkVpv(Vpv)
    if Vpv == 0
        result = 1;
    else
        result = 0;
    end
end

== matlab function 3_3PVstring/Subsystem6/MATLAB Function1 ==
  data: Vpv input; result output
function result = checkVpv(Vpv)
    if Vpv == 0
        result = 1;
    else
        result = 0;
    end
end

== matlab function 3_3PVstring/Subsystem7/MATLAB Function1 ==
  data: Vpv input; result output
function result = checkVpv(Vpv)
    if Vpv == 0
        result = 1;
    else
        result = 0;
    end
end

== matlab function 3_3PVstring/Subsystem8/MATLAB Function1 ==
  data: Vpv input; result output
function result = checkVpv(Vpv)
    if Vpv == 0
        result = 1;
    else
        result = 0;
    end
end
